simulink model "HW2LQR"  (R2021a)
settings: Solver=VariableStepAuto  StartTime=0.0  StopTime=20  RelTol=1e-3
settings Model: Creator=huangzijing  LastModifiedBy=huangzijing

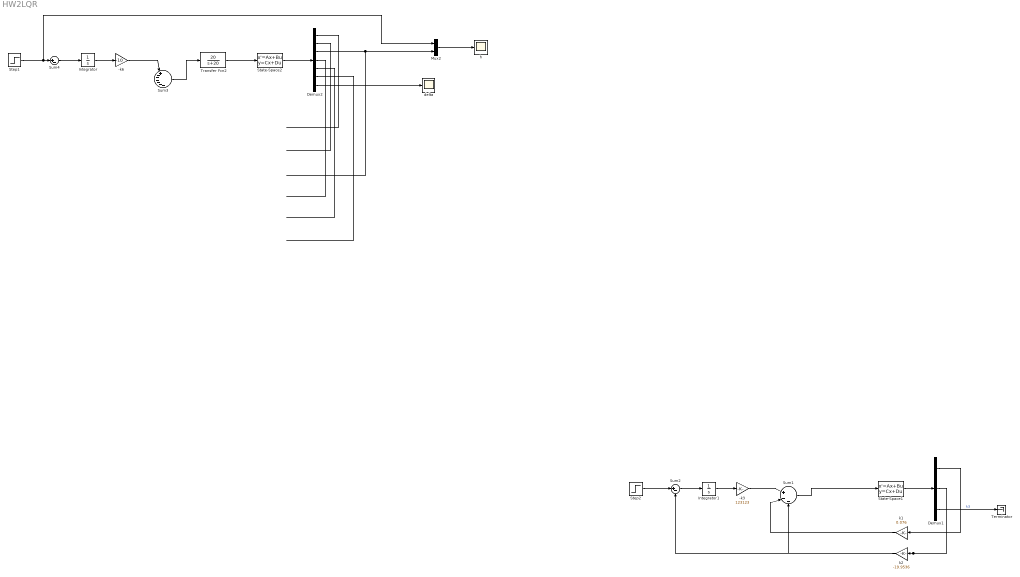
== system HW2LQR ==
  "-k3  " : Gain  Gain=123123
  "-k6  " : Gain  Gain=-10
  Demux1 : Demux  Outputs=3
  Demux2 : Demux  Outputs=7
  Integrator : Integrator
  Integrator1 : Integrator
  Mux2 : Mux  Inputs=2
  State-Space1 : StateSpace  A=|  B=[-0.0520;0.1016;0;0;116.3;0]  C=[1 0 0 0 0 0;0 1 0 0 0 0;0 0 1 0 0 0;0 0 0 1 0 0; 0 0 0 0 1 0;0 0 0 0 0 1;0 0 0 0 0 0 ]  D=[0;0;0;0;0;0;1]  InitialCondition=[50;0;100;0;0;0]
      | [-0.0064 9.2250 0 -9.8100 -0.8960 0;
      |     -0.0234 -5.1414 0 0 0.9519 0;
      |     0 25.000 0 -24.9836 0 0;
      |     0 0 0 0 1 0 ;
      |     0.7047 -485.6225 0 0 -31.4645 0;0 0 1 0 0 0]
  State-Space2 : StateSpace  A=|  B=[-0.0520;0.1016;0;0;116.3;0]  C=[1 0 0 0 0 0;0 1 0 0 0 0;0 0 1 0 0 0;0 0 0 1 0 0; 0 0 0 0 1 0;0 0 0 0 0 1;0 0 0 0 0 0 ]  D=[0;0;0;0;0;0;1]  InitialCondition=[50;0;100;0;0;0]
      | [-0.0064 9.2250 0 -9.8100 -0.8960 0;
      |     -0.0234 -5.1414 0 0 0.9519 0;
      |     0 25.000 0 -24.9836 0 0;
      |     0 0 0 0 1 0 ;
      |     0.7047 -485.6225 0 0 -31.4645 0;0 0 1 0 0 0]
  Step1 : Step  Before=100  After=200  SampleTime=0
  Step2 : Step  Before=100  After=200  SampleTime=0
  Sum1 : Sum  Inputs=|+--
  Sum2 : Sum  Inputs=|+-
  Sum3 : Sum  Inputs=|+------
  Sum4 : Sum  Inputs=|+-
  Terminator : Terminator
  Transfer Fcn2 : TransferFcn  Numerator=[20]  Denominator=[1 20]
  delta : Scope
  h : Scope
  k1 : Gain  Gain=0.076
  k2 : Gain  Gain=-19.9536
  wires:
  State-Space2/1 -> Demux2/1
  Demux2/3 -> Mux2/2
  Transfer Fcn2/1 -> State-Space2/1
  Mux2/1 -> h/1
  Demux2/1 -> ?
  Demux2/2 -> ?
  Demux2/4 -> ?
  Demux2/5 -> ?
  Demux2/6 -> ?
  Sum3/1 -> Transfer Fcn2/1
  "-k6  "/1 -> Sum3/1
  Integrator/1 -> "-k6  "/1
  Step1/1 -> Mux2/1, Sum4/1
  Sum4/1 -> Integrator/1
  Demux2/7 -> delta/1
  Demux1/1 -> k1/1
  Sum2/1 -> Integrator1/1
  Step2/1 -> Sum2/1
  "-k3  "/1 -> Sum1/1
  Integrator1/1 -> "-k3  "/1
  State-Space1/1 -> Demux1/1
  Demux1/2 -> Sum2/2, k2/1
  Sum1/1 -> State-Space1/1
  k2/1 -> Sum1/3
  k1/1 -> Sum1/2
  Demux1/3 -> Terminator/1  "k3"
